simulink model "servo_control"  (R2016b)
settings: Solver=FixedStepAuto  StartTime=0.0  StopTime=20  RelTol=1e-3  EnableMultiTasking=on
libraries: arduinolib x6
settings Model: ExtModeTrigDuration=2  Creator=root  LastModifiedBy=root
settings DataIOCC: ExternalInput=[xd]
settings OptimizationCC: MaxStackSize=64
settings DebuggingCC: ParameterTunabilityLossMsg=error
settings HardwareCC: ProdBitPerInt=16  ProdBitPerPointer=16  ProdBitPerSizeT=16  ProdBitPerPtrDiffT=16  ProdLargestAtomicFloat=None  ProdWordSize=8  ProdHWDeviceType=Atmel->AVR
settings RTWCC: SystemTargetFile=ert.tlc  HardwareBoard=Arduino Uno  TLCOptions=-aInlineSetEventsForThisBaseRateFcn=TLC_FALSE -aSuppressMultiTaskScheduler=TLC_FALSE -aRateBasedStepFcn=1  TemplateMakefile=ert_default_tmf  Description=Embedded Coder  GenerateReport=on  Toolchain=Arduino AVR  BuildConfiguration=Faster Runs  IncludeHyperlinkInReport=on  LaunchReport=on  GenerateTraceInfo=on  GenerateTraceReport=on  GenerateTraceReportSl=on  GenerateTraceReportSf=on  GenerateTraceReportEml=on
settings CodeAppCC: ForceParamTrailComments=on  IgnoreCustomStorageClasses=off  OperatorAnnotations=on  SimulinkDataObjDesc=on  SFDataObjDesc=on  MATLABFcnDesc=on  InsertBlockDesc=on  MATLABSourceComments=on
settings ERTTargetCC: SupportContinuousTime=on  SupportVariableSizeSignals=on

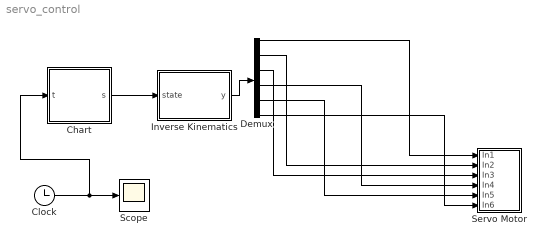
== system servo_control ==
  Chart : Stateflow chart  TreatAsAtomicUnit=on
  Clock : Clock
  Demux : Demux  Outputs=6
  Inverse Kinematics : MATLAB Function  TreatAsAtomicUnit=on
  Scope : Scope
  Servo Motor : Subsystem
  wires:
  Demux/1 -> Servo Motor/1(In1)
  Demux/2 -> Servo Motor/2(In2)
  Demux/3 -> Servo Motor/3(In3)
  Demux/4 -> Servo Motor/4(In4)
  Demux/5 -> Servo Motor/5(In5)
  Demux/6 -> Servo Motor/6(In6)
  Inverse Kinematics/1(y) -> Demux/1
  Chart/1(s) -> Inverse Kinematics/1(state)
  Clock/1 -> Chart/1(t), Scope/1

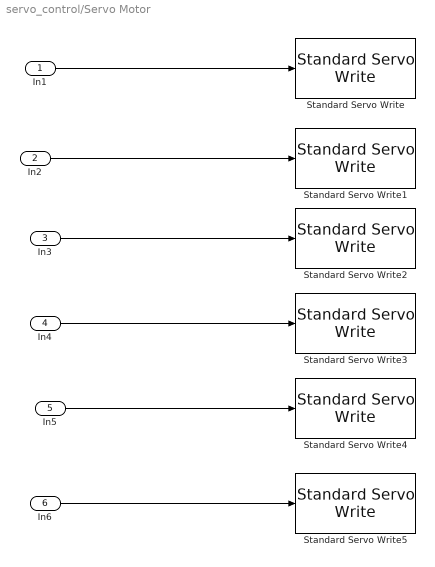
== system servo_control/Servo Motor ==
  In1 : Inport
  In2 : Inport  Port=2
  In3 : Inport  Port=3
  In4 : Inport  Port=4
  In5 : Inport  Port=5
  In6 : Inport  Port=6
  Standard Servo Write : arduinolib/Standard Servo Write  pinNumber=3  blockPlatform=arduino
  Standard Servo Write1 : arduinolib/Standard Servo Write  pinNumber=5  blockPlatform=arduino
  Standard Servo Write2 : arduinolib/Standard Servo Write  pinNumber=6  blockPlatform=arduino
  Standard Servo Write3 : arduinolib/Standard Servo Write  pinNumber=9  blockPlatform=arduino
  Standard Servo Write4 : arduinolib/Standard Servo Write  pinNumber=10  blockPlatform=arduino
  Standard Servo Write5 : arduinolib/Standard Servo Write  pinNumber=11  blockPlatform=arduino
  wires:
  In3/1 -> Standard Servo Write2/1
  In2/1 -> Standard Servo Write1/1
  In4/1 -> Standard Servo Write3/1
  In5/1 -> Standard Servo Write4/1
  In6/1 -> Standard Servo Write5/1
  In1/1 -> Standard Servo Write/1

== matlab function servo_control/Inverse Kinematics ==
  data: y output; state input
function y = Inv(state)
y=zeros(6,1);
S=coder.load('simu_xd');
if(state == 1)
    y=[S.qd;45];
else
    y=S.q0;
end
end

== stateflow chart servo_control/Chart ==
  state Reach
    entry: s=1;
    t2=t
  state Iniital
    entry: s = 0;
    t1=t;
  state End
    entry: s=2;
  (default) -> Iniital
  Iniital -> Reach : [(t-t1)>=5]
  Reach -> End : [(t-t2)>=5]
  data: s output; t input; t2 local; t1 local
